simulink model "Demo1202TTaskAssign"  (R2015b)
settings: Solver=ode1  StartTime=0.0  StopTime=Inf  FixedStep=0.001  RelTol=1e-3
PostLoadFcn:
  | , if any(exist('dsrtsu_mdlpostloadfcn', 'file') == [2, 3, 6]), try dsrtsu_mdlpostloadfcn('Execute', bdroot); catch fprintf('Error in PostLoadFcn (dsrtsu_mdlpostloadfcn) for model "%s":\n %s\n', bdroot, lasterr); end, end,
libraries: RTITaskLibDemoLibInfo x4, rti1202lib_dio_class1 x2, rtitasklib x1
settings Model: DSRTSU_INTERNAL_RTI_VER=500  DSRTSU_INTERNAL_RTI_TYPE=rti1202  RTICANMMDATA=struct('GeneralSetupData',struct('modelroot',['L:\New folder\REC_Maroje\Demo1\RTI\Demos\Model\TaskLib\Model\TTaskAssign'],'generalsettings',struct('filesettings',struct('destfolder',struct('Name','RTICANMM_FILES','Check',1),'buildfolder',struct('Name','.','Check',1),'AbsDestfolder',struct('Name',['L:\New folder\REC_Maroje\Demo1\RTI\Demos\Model\TaskLib\Model\TTaskAssign\RTICANMM_FILES']),'AbsBuildfolder',struct('Name',['L:\New folder\REC_Maroje\Demo1\RTI\Demos\Model\TaskLib\Model\TTaskAssign']))),'options',struct('addpaths',1,'rmpaths',1,'addtrcexclusion',logical(1),'cannavigator',struct('checkmonitoring',0),'show_usrtrc',0,'use_usrtrc',0),'advanced',struct('options',ones(1,100)),'MPSetup',{{}},'modelname','Demo1202TTaskAssign','block','Demo1202TTaskAssign'))  DSRTSU_INTERNAL_RTIFLEXRAYCONFIG=110  DSRTSU_INTERNAL_RTIFPGA=90  Creator=dSPACE GmbH  LastModifiedBy=dSPACE GmbH
settings DataIOCC: SaveFormat=Array  SignalLoggingSaveFormat=ModelDataLogs
settings OptimizationCC: BlockReduction=off  ConditionallyExecuteInputs=off  OptimizeBlockIOStorage=off  BufferReuse=off  GlobalBufferReuse=off  ExpressionFolding=off  ExpressionDepthLimit=2147483647  LocalBlockOutputs=off  InitFltsAndDblsToZero=on
settings DebuggingCC: SaveWithParameterizedLinksMsg=none  UnderspecifiedInitializationDetection=Classic  MergeDetectMultiDrivingBlocksExec=none  SignalResolutionControl=TryResolveAllWithWarning  SolverPrmCheckMsg=warning  MultiTaskDSMMsg=warning  MultiTaskCondExecSysMsg=none  MultiTaskRateTransMsg=warning  TasksWithSamePriorityMsg=none  FcnCallInpInsideContextMsg=UseLocalSettings  StateNameClashWarn=warning  StrictBusMsg=None
settings HardwareCC: ProdBitPerPointer=32  ProdLargestAtomicInteger=Integer  ProdEndianess=BigEndian  ProdWordSize=32  ProdHWDeviceType=Custom Processor->Custom  TargetIntDivRoundTo=Zero  TargetEndianess=BigEndian  TargetHWDeviceType=Custom Processor->Custom
settings RTWCC: SystemTargetFile=rti1202.tlc  MakeCommand=make_rti  TemplateMakefile=rti1202.tmf  Description=dSPACE DS1202 Hardware Platform  RTWVerbose=off
settings STFCustomTargetCC: ParMdlRefBuildCompliant=on  ConcurrentExecutionCompliant=off  GeneratePreprocessorConditionals=Use local settings  CPPClassGenCompliant=off  GRTInterface=off  SystemTargetFile=rti1202.tlc
settings GRTTargetCC: CompOptLevelCompliant=off  ConcurrentExecutionCompliant=off  CombineOutputUpdateFcns=off  MatFileLogging=off  CPPClassGenCompliant=off  UseToolchainInfoCompliant=off  ExtModeMexFile=noextcomm
settings ConfigComp: CovModelRefEnable=Off

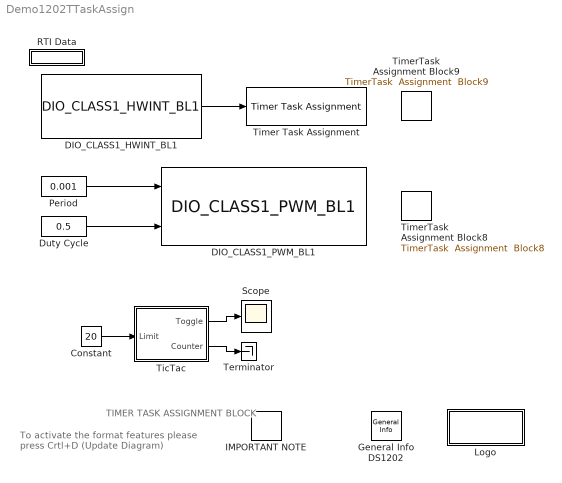
== system Demo1202TTaskAssign ==
  note: To activate the format features please
      | press Crtl+D (Update Diagram)
  note: TIMER TASK ASSIGNMENT BLOCK
  Constant : Constant  Value=20
  DIO_CLASS1_HWINT_BL1 : rti1202lib_dio_class1/DIO_CLASS1_HWINT_BL1  DSProperties=struct('RTI',struct('Version',uint32(2),'BlockType',struct('isSLSource',uint8(1),'isSLSink',uint8(0),'isHWSource',uint8(0),'isHWSink',uint8(0),'isSetup',uint8(0),'isInline',uint8(1),'isNonInline',uint8(0),'isInterrupt',uint8(1),'isChannelwise',uint8(0)),'IOBoardType',{{'DS120X','STD','DIOC1'}},'UnitType','DSTASKTOOL','Identifier','HWINT','DialogType','ML','BlockSet','NONE','SlaveProcessor','NONE'))  RTIBlockInterface=struct('OutputPortsActive',1,'OutputPortsWidth',int32(1),'OutputPortsName',{{'Interrupt'}},'FunctionCall',uint32(0),'DialogFcn','rti120xstddioc1hwintgui','InitLevel',3,'BlockDisplay',{{['DIO CL1 HWINT\nPort: 1\nChannel: 1'],'center'}},'IconTransparency','on','BlockName',struct('Token',{{'DIO_CLASS1_HWINT_BL1'}}))  RTIBlockParameters=struct('SourceBlockListIdx',{{2,'OFF',[1 2]}},'SourceBlockIdentifier',{{'PWM','OFF',[]}},'InterruptTypeListIdx',{{2,'OFF',[1 2]}},'InterruptType',{{['Falling edge'],'OFF',[]}},'PortNo',{{1,'OFF',[]}},'ChannelNo',{{1,'OFF',[]}})  RTISFcnParameters=struct('PortNo','int16','ChannelNo','int16')  RTIBlockParaDefault=struct('SourceBlockListIdx',1,'SourceBlockIdentifier',['NOT SELECTED'],'InterruptTypeListIdx',1,'InterruptType',['NOT SELECTED'],'PortNo',-1,'ChannelNo',-1)
  DIO_CLASS1_PWM_BL1 : rti1202lib_dio_class1/DIO_CLASS1_PWM_BL1  DSProperties=struct('RTI',struct('Version',uint32(1),'BlockType',struct('isSLSource',uint8(0),'isSLSink',uint8(1),'isHWSource',uint8(0),'isHWSink',uint8(1),'isSetup',uint8(0),'isInline',uint8(1),'isNonInline',uint8(0),'isInterrupt',uint8(0),'isChannelwise',uint8(1)),'IOBoardType',{{'DS120X','STD','DIOC1'}},'UnitType','PWM','Identifier','PWM','DialogType','ML','BlockSet','NONE','SlaveProcessor','NONE'))  RTIBlockInterface=struct('InputPortsWidth',int32([1 1]),'InputPortsActive',[1 1],'InputPortsName',{{'Period',['Duty Cycle']}},'BlockDisplay',{{['DIO CL1 PWM\nPort: 1\nChannel: 1'],'center'}},'IconTransparency','on','InitLevel',3,'DialogFcn','rti120xstddioc1pwmgui','BlockName',struct('Token',{{'DIO_CLASS1_PWM_BL1'}}))  RTIBlockParameters=struct('PortNo',{{1,'OFF',[]}},'ChannelNo',{{1,'OFF',[]}},'HighLevel',{{1,'OFF',[1 3]}},'UpdateMode',{{2,'OFF',[1 2]}},'InvertingMode',{{1,'OFF',[1 2]}},'DutyCycleInit',{{'0.5','OFF',[0 1]}},'DutyCycleTerm',{{'0.5','OFF',[0 1]}},'PeriodInit',{{'5e-05','OFF',[1e-7 1.34]}},'PeriodTerm',{{'5e-05','OFF',[1e-7 1.34]}},'TerminationMode',{{0,'OFF',[0 1]}},'OutputTermValidate',{{0,'OFF',[0 1]}},'OutputTermBuildCheck',{{logical(0),'OFF',[]}},'EnableEvent',{{1,'OFF',[0 1]}},'EventMode',{{1,'OFF',[1 3]}},'EventOnFalling',{{1,'OFF',[0 1]}},'EventOnRising',{{0,'OFF',[0 1]}},'EventDelay',{{'0','OFF',[0 1.34]}},'EventRate',{{'1','OFF',[1 256]}},'EventBuildCheck',{{logical(1),'OFF',[]}},'TriggerLine',{{1,'OFF',[1 16]}},'TLCFileName',{{'rti120xdio_c1_pwm','OFF',[]}})  RTISFcnParameters=struct('PortNo','int16','ChannelNo','int16','HighLevel','int16','UpdateMode','int16','InvertingMode','int16','DutyCycleInit','double','DutyCycleTerm','double','PeriodInit','double','PeriodTerm','double','TerminationMode','int16','OutputTermValidate','int16','EnableEvent','int16','EventMode','int16','EventOnFalling','int16','EventOnRising','int16','EventDelay','double','EventRate','int16','TriggerLine','int16','TLCFileName','char')  RTIBlockParaDefault=struct('PortNo',1,'ChannelNo',1,'HighLevel',1,'UpdateMode',1,'InvertingMode',1,'DutyCycleInit',2^-1,'DutyCycleTerm',2^-1,'PeriodInit',5e-5,'PeriodTerm',5e-5,'TerminationMode',0,'OutputTermValidate',0,'OutputTermBuildCheck',0,'EnableEvent',0,'EventMode',1,'EventOnFalling',1,'EventOnRising',0,'EventDelay',0,'EventRate',1,'EventBuildCheck',0,'TriggerLine',1,'TLCFileName','rti120xdio_c1_pwm')
  Duty Cycle : Constant  Value=0.5
  General Info DS1202 : RTITaskLibDemoLibInfo/General Info  SystemSampleTime=-1
  IMPORTANT NOTE : RTITaskLibDemoLibInfo/IMPORTANT NOTE  SystemSampleTime=-1
  Logo : Subsystem  mask(dSPACE){EmptyParameter=[]}
      mask prompts: EmptyParameter "Mask Parameter 1:"
      settings: OpenFcn=;
      mask Display: image(imread('rti_mdl_dslogo.tif'));
  Period : Constant  Value=0.001
  RTI Data : Subsystem  Tag=struct('RTIDataServer',struct('RTIDataServerVs','2','RTIModelDescription','struct(''main'',''Demo1202TTaskAssign'',''sub'','''',''isMp'',0)'))  LoadFcn="if exist('rtidc'), try,  rtidc('DataHostBlockClbLoad', gcbh); catch, disp(['Warning: ''LoadFcn'' for RTI Data block failed: ' lasterr]); end, end,"  mask(RTI_DATA_HOST){}
      mask help:
      | RTI Data Block.
      | This block is used by RTI to store internal model-dependent data.
      | Please keep this block on the root level of the model. Deleting this block will result in data loss.
      |
      | NEVER DELETE OR COPY THIS BLOCK!
      settings: CopyFcn="if exist('rtidc'), try,  rtidc('DataHostBlockClbCopy', gcbh); catch, disp(['Warning: ''CopyFcn'' for RTI Data block failed: ' lasterr]); end, end,"  DeleteFcn="if exist('rtidc'), try,  rtidc('DataHostBlockClbDelete', gcbh); catch, disp(['Warning: ''DeleteFcn'' for RTI Data block failed: ' lasterr]); end, end,"  ModelCloseFcn="if exist('rtidc'), try,  rtidc('DataHostBlockClbModelClose', gcbh); catch, disp(['Warning: ''ModelCloseFcn'' for RTI Data block failed: ' lasterr]); end, end,"  PreSaveFcn="if exist('rtidc'), try,  rtidc('DataHostBlockClbPreSave', gcbh); catch, disp(['Warning: ''PreSaveFcn'' for RTI Data block failed: ' lasterr]); end, end,"  PostSaveFcn="if exist('rtidc'), try,  rtidc('DataHostBlockClbPostSave', gcbh); catch, disp(['Warning: ''PostSaveFcn'' for RTI Data block failed: ' lasterr]); end, end,"  NameChangeFcn="if exist('rtidc'), try,  rtidc('DataHostBlockClbNameChange', gcbh); catch, disp(['Warning: ''NameChangeFcn'' for RTI Data block failed: ' lasterr]); end, end,"
      mask Help:
      | RTI Data Block.
      | This block is used by RTI to store internal model-dependent data.
      | Please keep this block on the root level of the model. Deleting this block will result in data loss.
      | 
      | NEVER DELETE OR COPY THIS BLOCK!
      mask Display:
      | text(0.5, 0.5, 'RTI Data', 'HorizontalAlignment', 'center');
      | plot([1 0]);
  Scope : Scope
  Terminator : Terminator
  TicTac : Subsystem
      mask help:
      | The output "Toggle" changes its output between -1 and 1 each time the block is executed.
      |
      | The output "Counter" counts up to the given "Limit" and then resets to one.
  Timer Task Assignment : rtitasklib/Timer Task Assignment  Reserved2=[]  Reserved3=[]  Reserved4=[]  DSProperties=struct('RTI',struct('Version',uint32(2),'BlockType',struct('isSLSource',uint8(0),'isSLSink',uint8(1),'isHWSource',uint8(0),'isHWSink',uint8(0),'isSetup',uint8(0),'isInline',uint8(1),'isNonInline',uint8(0),'isInterrupt',uint8(0),'isChannelwise',uint8(0)),'IOBoardType','INTLIB','UnitType','TTASSIGN','Identifier','TTASSIGN','DialogType','SL','BlockSet','NONE','SlaveProcessor','NONE','RelationId',struct('TH',struct('BlockId','TTASSIGN'))))
  TimerTask Assignment Block8 : RTITaskLibDemoLibInfo/TimerTask  Assignment  Block8  SystemSampleTime=-1
  TimerTask Assignment Block9 : RTITaskLibDemoLibInfo/TimerTask  Assignment  Block9  SystemSampleTime=-1
  wires:
  DIO_CLASS1_HWINT_BL1/1 -> Timer Task Assignment/1
  Duty Cycle/1 -> DIO_CLASS1_PWM_BL1/2
  Period/1 -> DIO_CLASS1_PWM_BL1/1
  Constant/1 -> TicTac/1(Limit)
  TicTac/2(Counter) -> Terminator/1
  TicTac/1(Toggle) -> Scope/1

== system Demo1202TTaskAssign/Logo ==
  note: $RCSfile: Demo1401TTaskAssign.mdl $
  note: $Date: 2012/07/16 15:49:30MESZ $
  note: $Revision: 2.3 $

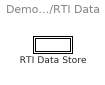
== system Demo1202TTaskAssign/RTI Data ==
  RTI Data Store : Subsystem  Tag="struct('private',struct('version',struct('dsVer',uint32(2),'dsVerCreation',uint32(2),'RTI',struct('ver','X.Y.Z','type','RTI1005')),'access',struct('type','Model','isPerm',1,'created',['16-Feb-2001 13:45:51'],'modified',['03-Feb-2017 15:09:09'],'location','')),'public',struct('main',struct('data',[]),'sub',struct('name',{{'Demo1202TTaskAssign'}},'data',{{struct('TH',struct('thTaskInfo',struct('taskType',{'TIMER','HWINT','TMRINT','SWINT','GLINT'},'tasksNumOf',{1,0,0,0,0},'srcIds',{{'120XDIOCL1PWM_FALLING_EDGEP1Ch1'},{},{},{},{}},'taskNames',{{['Timer Task 1']},{},{},{},{}})),'th_tc',struct('dataType','TASK','taskGroupId','','taskGroupList',{{}},'taskSchedulingPolicy','FCFS','taskType','TIMER','blkh',['Demo1202TTaskAssign/DIO_CLASS1_HWINT_BL1/Common Hardware' char(10) 'Interrupt Interface'],'srcId','120XDIOCL1PWMIntT2P1Ch1','srcSgnName',['DIO Type CL1 PWM Port 1 Channel 1 Falling edge'],'srcCpuName','','taskName',['Timer Task 1  [0.001] s'],'taskNameDisplayExt','','smplTime',0.001,'smplTimeOffs',0,'hasFixedPriority',0,'priority',1,'hasFixedOvc',0,'ovcType',1,'ovcMax',0),'tc_th',struct('dataType','TASK','taskGroupId','','taskGroupList',{{}},'taskSchedulingPolicy','FCFS','taskType','TIMER','blkh',['Demo1202TTaskAssign/DIO_CLASS1_HWINT_BL1/Common Hardware' char(10) 'Interrupt Interface'],'srcId','120XDIOCL1PWM_FALLING_EDGEP1Ch1','srcSgnName',['DIO Type CL1 PWM Port 1 Channel 1 Falling edge'],'srcCpuName','','taskName',['Timer Task 1  [0.001] s'],'taskNameDisplayExt','','smplTime',0.001,'smplTimeOffs',0,'hasFixedPriority',0,'priority',1,'hasFixedOvc',0,'ovcType',1,'ovcMax',0))}})))"  mask(RTI_DATA_STORE){}
      mask help:
      | RTI Data Store Block. This block is used by RTI to store internal model dependent data. Deleting this block will result in data loss.
      |
      | NEVER DELETE, COPY, OR MODIFY THIS BLOCK!
      mask Help:
      | RTI Data Store Block. This block is used by RTI to store internal model dependent data. Deleting this block will result in data loss.
      | 
      | NEVER DELETE, COPY, OR MODIFY THIS BLOCK!
      mask Display: text(0.5, 0.5, ' ', 'HorizontalAlignment', 'center');

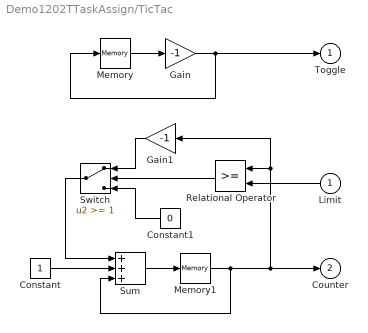
== system Demo1202TTaskAssign/TicTac ==
  Limit : Inport
  Constant : Constant
  Constant1 : Constant  Value=0
  Gain : Gain  Gain=-1  SaturateOnIntegerOverflow=on  OutDataTypeStr=Inherit: Same as input  ParamDataTypeStr=Inherit: Same as input
  Gain1 : Gain  Gain=-1  SaturateOnIntegerOverflow=on  OutDataTypeStr=Inherit: Same as input  ParamDataTypeStr=Inherit: Same as input
  Memory : Memory  X0=-1  InheritSampleTime=on
  Memory1 : Memory  InheritSampleTime=on
  Relational Operator : RelationalOperator  InputSameDT=on
  Sum : Sum  Inputs=+++  SaturateOnIntegerOverflow=on  InputSameDT=on  OutDataTypeStr=Inherit: Same as first input
  Switch : Switch  Threshold=1  SaturateOnIntegerOverflow=on  InputSameDT=on
  Toggle : Outport
  Counter : Outport  Port=2
  wires:
  Constant1/1 -> Switch/3
  Gain1/1 -> Switch/1
  Switch/1 -> Sum/1
  Constant/1 -> Sum/2
  Sum/1 -> Memory1/1
  Gain/1 -> Toggle/1, Memory/1
  Memory/1 -> Gain/1
  Relational Operator/1 -> Switch/2
  Limit/1 -> Relational Operator/2
  Memory1/1 -> Counter/1, Relational Operator/1, Gain1/1, Sum/3

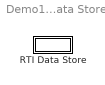
== system Demo1202TTaskAssign/RTI Data/RTI Data Store ==
  RTI Data Store : Subsystem  mask(RTI_DATA_STORE){}
      mask help:
      | RTI Data Store Block. This block is used by RTI to store internal model dependent data. Deleting this block will result in data loss.
      |
      | NEVER DELETE, COPY, OR MODIFY THIS BLOCK!
      mask Help:
      | RTI Data Store Block. This block is used by RTI to store internal model dependent data. Deleting this block will result in data loss.
      | 
      | NEVER DELETE, COPY, OR MODIFY THIS BLOCK!
      mask Display: text(0.5, 0.5, ' ', 'HorizontalAlignment', 'center');

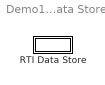
== system Demo1202TTaskAssign/RTI Data/RTI Data Store/RTI Data Store ==
  RTI Data Store : Subsystem  mask(RTI_DATA_STORE){}
      mask help:
      | RTI Data Store Block. This block is used by RTI to store internal model dependent data. Deleting this block will result in data loss.
      |
      | NEVER DELETE, COPY, OR MODIFY THIS BLOCK!
      mask Help:
      | RTI Data Store Block. This block is used by RTI to store internal model dependent data. Deleting this block will result in data loss.
      | 
      | NEVER DELETE, COPY, OR MODIFY THIS BLOCK!
      mask Display: text(0.5, 0.5, ' ', 'HorizontalAlignment', 'center');

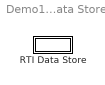
== system Demo1202TTaskAssign/RTI Data/RTI Data Store/RTI Data Store/RTI Data Store ==
  RTI Data Store : Subsystem  mask(RTI_DATA_STORE){}
      mask help:
      | RTI Data Store Block. This block is used by RTI to store internal model dependent data. Deleting this block will result in data loss.
      |
      | NEVER DELETE, COPY, OR MODIFY THIS BLOCK!
      mask Help:
      | RTI Data Store Block. This block is used by RTI to store internal model dependent data. Deleting this block will result in data loss.
      | 
      | NEVER DELETE, COPY, OR MODIFY THIS BLOCK!
      mask Display: text(0.5, 0.5, ' ', 'HorizontalAlignment', 'center');

== system Demo1202TTaskAssign/RTI Data/RTI Data Store/RTI Data Store/RTI Data Store/RTI Data Store ==
